simulink model "attack_decay_filter_sim"  (R2020b)
settings: Solver=VariableStepAuto  StartTime=0.0  StopTime=stopTime  RelTol=1e-3
InitFcn:
  | initCallback
StopFcn:
  | stopCallback
undefined symbols (not defined in the file or in its folder): attack_c1_a, attack_c2_a, decay_c1_r, decay_c2_r, mp
settings Model: Creator=t96f346  LastModifiedBy=conno
settings DataIOCC: ReturnWorkspaceOutputs=off

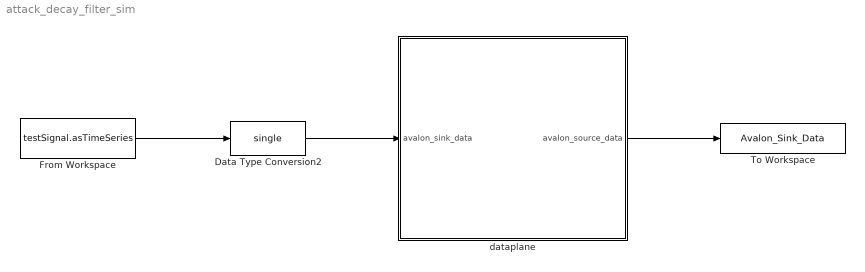
== system attack_decay_filter_sim ==
  Data Type Conversion2 : DataTypeConversion  OutDataTypeStr=single  RndMeth=Nearest
  From Workspace : FromWorkspace  VariableName=testSignal.asTimeSeries  SampleTime=mp.Ts
  To Workspace : ToWorkspace  VariableName=Avalon_Sink_Data  SampleTime=-1
  dataplane : Subsystem  TreatAsAtomicUnit=on
  wires:
  Data Type Conversion2/1 -> dataplane/1(avalon_sink_data)
  From Workspace/1 -> Data Type Conversion2/1
  dataplane/1(avalon_source_data) -> To Workspace/1

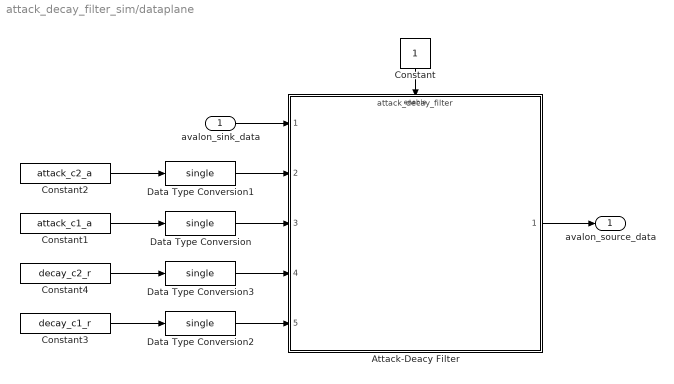
== system attack_decay_filter_sim/dataplane ==
  avalon_sink_data : Inport
  Attack-Deacy Filter : ModelReference  ModelNameDialog=attack_decay_filter  SimulationMode=Normal  ModelReferenceVersion=2.61  EnablePortName=Enable  EnablePortStatesWhenEnabling=held
  Constant : Constant  OutDataTypeStr=boolean  SampleTime=-1
  Constant1 : Constant  Value=attack_c1_a  SampleTime=-1
  Constant2 : Constant  Value=attack_c2_a  SampleTime=-1
  Constant3 : Constant  Value=decay_c1_r  SampleTime=-1
  Constant4 : Constant  Value=decay_c2_r  SampleTime=-1
  Data Type Conversion{,1..3} (4 alike) : DataTypeConversion  OutDataTypeStr=single  RndMeth=Nearest
  avalon_source_data : Outport  VectorParamsAs1DForOutWhenUnconnected=off
  wires:
  avalon_sink_data/1 -> Attack-Deacy Filter/1
  Data Type Conversion1/1 -> Attack-Deacy Filter/2
  Constant4/1 -> Data Type Conversion3/1
  Constant2/1 -> Data Type Conversion1/1
  Data Type Conversion3/1 -> Attack-Deacy Filter/4
  Attack-Deacy Filter/1 -> avalon_source_data/1
  Constant/1 -> Attack-Deacy Filter/Enable
  Data Type Conversion/1 -> Attack-Deacy Filter/3
  Constant1/1 -> Data Type Conversion/1
  Data Type Conversion2/1 -> Attack-Deacy Filter/5
  Constant3/1 -> Data Type Conversion2/1
